simulink model "simulation_control_observerLQR_L_WP3"  (R2023b)
settings: Solver=VariableStepAuto  StartTime=0.0  StopTime=10.0  RelTol=1e-3
values from neighbouring files (symbols this model uses):
  A = [0 1; 9.81 -0.1]    [WP3.m]
  B = [0; 1]    [WP3.m]
  C = [1 0]    [WP3.m]
  K = [92.0469   14.4179]    [WP3.m]
  L = [l1; l2]    [WP3.m]
settings Model: Creator=giova  LastModifiedBy=giova

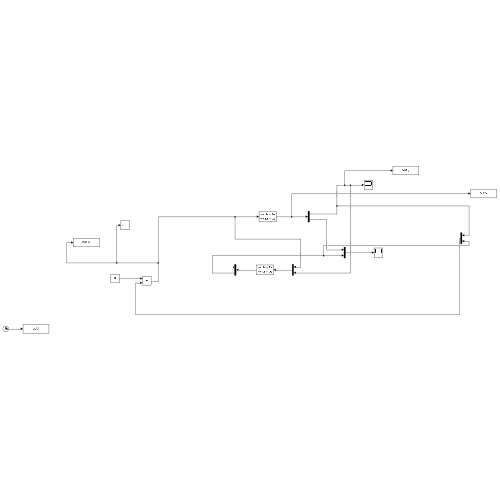
[thumbnail: Simulink's stored preview of the top-level diagram]
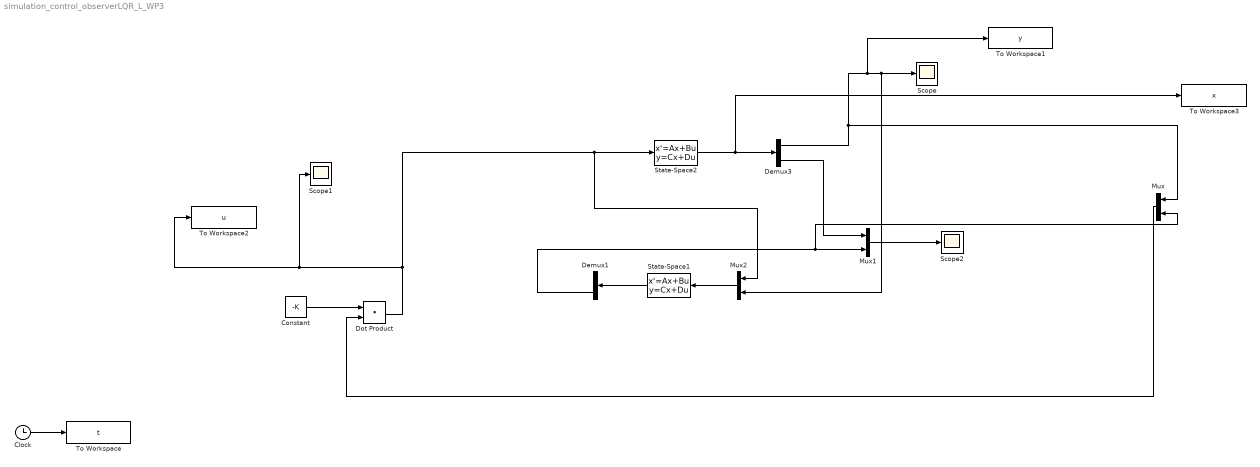
== system simulation_control_observerLQR_L_WP3 ==
  Clock : Clock
  Constant : Constant  Value=-K
  Demux1 : Demux  Outputs=2
  Demux3 : Demux  Outputs=2
  Dot Product : DotProduct  OutDataTypeStr=Inherit: Inherit via internal rule
  Mux : Mux  Inputs=2
  Mux1 : Mux  Inputs=2
  Mux2 : Mux  Inputs=2
  Scope : Scope
  Scope1 : Scope
  Scope2 : Scope
  State-Space1 : StateSpace  A=A-L*C  B=[B L]  C=eye(2)  D=[0 0; 0 0]  InitialCondition=[0 0]
  State-Space2 : StateSpace  A=A  B=B  C=eye(2)  D=[0 ; 0]  InitialCondition=[pi 0]
  To Workspace : ToWorkspace  VariableName=t  SampleTime=-1
  To Workspace1 : ToWorkspace  VariableName=y  SampleTime=-1
  To Workspace2 : ToWorkspace  VariableName=u  SampleTime=-1
  To Workspace3 : ToWorkspace  VariableName=x  SampleTime=-1
  wires:
  Dot Product/1 -> Mux2/1, State-Space2/1, To Workspace2/1, Scope1/1
  Constant/1 -> Dot Product/1
  Clock/1 -> To Workspace/1
  Demux1/2 -> Mux/2, Mux1/2
  Mux1/1 -> Scope2/1
  State-Space1/1 -> Demux1/1
  State-Space2/1 -> To Workspace3/1, Demux3/1
  Demux3/1 -> Mux/1, To Workspace1/1, Mux2/2, Scope/1
  Mux2/1 -> State-Space1/1
  Mux/1 -> Dot Product/2
  Demux3/2 -> Mux1/1
